simulink model "comunicationUDP_2015"  (Simulink 8.5)
settings: Solver=ode3  SolverMode=SingleTasking  StartTime=0.0  StopTime=inf  FixedStep=0.01  RelTol=1e-3
undefined symbols (not defined in the file or in its folder): get, hot
libraries: mblibv1 x4, dspnetwork x2, etargetslib x1, vrlib x1, dspsnks4 x1
settings Model: Creator=zigg  LastModifiedBy=nakano  CovMetricSettings=dwe  CovHtmlReporting=off  covSaveCumulativeToWorkspaceVar=off  CovSaveSingleToWorkspaceVar=off  CovExternalEMLEnable=on
settings DataIOCC: LimitDataPoints=off  SaveFormat=Dataset  SignalLoggingSaveFormat=Dataset
settings OptimizationCC: ExpressionDepthLimit=128
settings DebuggingCC: UnderspecifiedInitializationDetection=Simplified  MergeDetectMultiDrivingBlocksExec=error  FcnCallInpInsideContextMsg=EnableAllAsError  StateNameClashWarn=none  SFUnexpectedBacktrackingDiag=error  SFNoUnconditionalDefaultTransitionDiag=error
settings HardwareCC: ProdBitPerPointer=64  ProdLargestAtomicFloat=Float  ProdIntDivRoundTo=Zero  ProdEndianess=LittleEndian  ProdHWDeviceType=Specified
settings ModelReferenceCC: PropagateSignalLabelsOutOfModel=on
settings GRTTargetCC: TargetLangStandard=C99 (ISO)  GeneratePreprocessorConditionals=Use local settings  CombineOutputUpdateFcns=on  GRTInterface=off

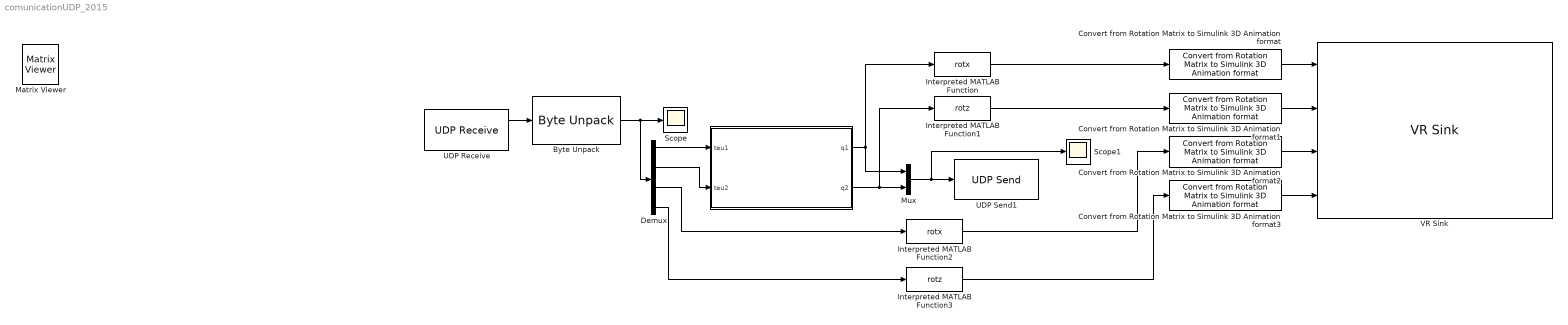
== system comunicationUDP_2015 ==
  "  " : Subsystem
  Byte Unpack : etargetslib/Byte Unpack  dimensions={[4]}  datatypes={'double'}  byteAlign=1
  Convert from Rotation Matrix to Simulink 3D Animation format{,1..3} (4 alike) : mblibv1/Utilities/Convert from Rotation Matrix to Simulink 3D Animation format
  Demux : Demux
  Interpreted MATLAB Function : MATLABFcn  MATLABFcn=rotx
  Interpreted MATLAB Function1 : MATLABFcn  MATLABFcn=rotz
  Interpreted MATLAB Function2 : MATLABFcn  MATLABFcn=rotx
  Interpreted MATLAB Function3 : MATLABFcn  MATLABFcn=rotz
  Mux : Mux  Inputs=2
  Scope : Scope
      settings: YMin=-110.65543  YMax=995.8989
  Scope1 : Scope
      settings: YMin=-110.65543  YMax=995.8989
  UDP Receive : dspnetwork/UDP Receive  localURL='0.0.0.0'  localPort=4000  remoteURL='192.168.2.239'  remotePort=-1  recvBufferSize=8192  dims=32  signalDatatype=uint8  isVarSize=off  showBlockingTime=off  blockingTime=0  sampletime=0.01  blockPlatform=[]
  UDP Send1 : dspnetwork/UDP Send  remoteURL='192.168.2.239'  remotePort=4000  localURL='0.0.0.0'  localPortSource=Automatically determine  localPort=-1  sampletime=-1  blockPlatform=[]  separateLengthPort=0
  VR Sink : vrlib/VR Sink  InstantiateOnLoad=on  SampleTime=0.1  ViewEnable=on  RemoteChange=off  RemoteView=off  FieldsWritten=Joint1.rotation.4.1.1.double#Joint2.rotation.4.1.1.double#Joint1_SP.rotation.4.1.1.double#Joint2_SP.rotation.4.1.1.double  WorldFileName=my_robot.wrl  AutoView=off  VideoDimensions=[]  AllowVariableSize=off
  Matrix Viewer : dspsnks4/Matrix Viewer  IOType=viewer  ImageParams=off  CMapStr=hot(256)  AxisColorbar=on  AxisParams=off  AxisOrigin=Upper left corner  XLabel=X-axis  YLabel=Y-axis  ZLabel=Z-axis  FigPos=get(0,'defaultfigureposition')  AxisZoom=off
      settings: YMin=-1.0  YMax=1.0
  wires:
  UDP Receive/1 -> Byte Unpack/1
  Byte Unpack/1 -> Demux/1, Scope/1
  Demux/1 -> "  "/1(tau1)
  Demux/2 -> "  "/2(tau2)
  Mux/1 -> UDP Send1/1, Scope1/1
  "  "/1(q1) -> Mux/1, Interpreted MATLAB Function/1
  "  "/2(q2) -> Interpreted MATLAB Function1/1, Mux/2
  Interpreted MATLAB Function/1 -> Convert from Rotation Matrix to Simulink 3D Animation format/1
  Interpreted MATLAB Function1/1 -> Convert from Rotation Matrix to Simulink 3D Animation format1/1
  Interpreted MATLAB Function2/1 -> Convert from Rotation Matrix to Simulink 3D Animation format2/1
  Demux/3 -> Interpreted MATLAB Function2/1
  Demux/4 -> Interpreted MATLAB Function3/1
  Convert from Rotation Matrix to Simulink 3D Animation format/1 -> VR Sink/1
  Convert from Rotation Matrix to Simulink 3D Animation format1/1 -> VR Sink/2
  Convert from Rotation Matrix to Simulink 3D Animation format2/1 -> VR Sink/3
  Interpreted MATLAB Function3/1 -> Convert from Rotation Matrix to Simulink 3D Animation format3/1
  Convert from Rotation Matrix to Simulink 3D Animation format3/1 -> VR Sink/4

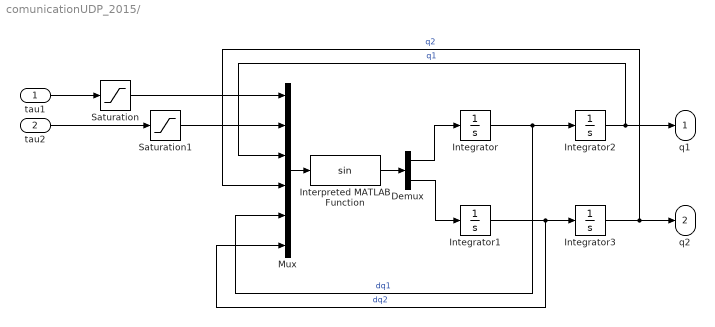
== system comunicationUDP_2015/   ==
  tau1 : Inport
  tau2 : Inport  Port=2
  Demux : Demux  Outputs=2
  Integrator : Integrator
  Integrator1 : Integrator
  Integrator2 : Integrator  InitialCondition=pi/2*0
  Integrator3 : Integrator  InitialCondition=1.87*0
  Interpreted MATLAB Function : MATLABFcn
  Mux : Mux  Inputs=6
  Saturation : Saturate  UpperLimit=1.18  LowerLimit=-1.18
  Saturation1 : Saturate  UpperLimit=1.18  LowerLimit=-1.18
  q1 : Outport  PortDimensions=1
  q2 : Outport  Port=2  PortDimensions=1
  wires:
  Demux/1 -> Integrator/1
  Demux/2 -> Integrator1/1
  Integrator1/1 -> Mux/6, Integrator3/1  "dq2"
  Integrator2/1 -> Mux/3, q1/1  "q1"
  Integrator3/1 -> Mux/4, q2/1  "q2"
  Integrator/1 -> Mux/5, Integrator2/1  "dq1"
  tau1/1 -> Saturation/1
  tau2/1 -> Saturation1/1
  Saturation/1 -> Mux/1
  Saturation1/1 -> Mux/2
  Mux/1 -> Interpreted MATLAB Function/1
  Interpreted MATLAB Function/1 -> Demux/1
